simulink model "lsys1"  (R2020b)
settings: Solver=VariableStepAuto  StartTime=0.0  StopTime=10.0  RelTol=1e-3
settings Model: Creator=반달  LastModifiedBy=반달

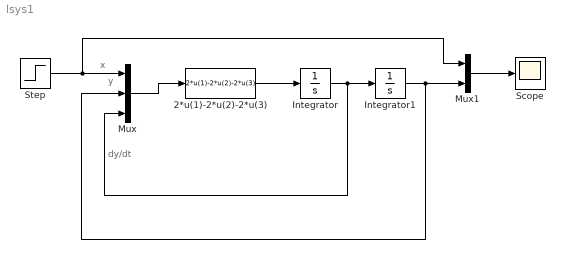
== system lsys1 ==
  note: dy/dt
  note: y
  note: x
  2*u(1)-2*u(2)-2*u(3) : MATLABFcn  MATLABFcn=2*u(1)-2*u(2)-2*u(3)
  Integrator : Integrator
  Integrator1 : Integrator
  Mux : Mux  Inputs=3
  Mux1 : Mux  Inputs=2
  Scope : Scope
  Step : Step  Time=0  SampleTime=0
  wires:
  Step/1 -> Mux1/1, Mux/1
  Mux/1 -> 2*u(1)-2*u(2)-2*u(3)/1
  2*u(1)-2*u(2)-2*u(3)/1 -> Integrator/1
  Integrator/1 -> Mux/3, Integrator1/1
  Integrator1/1 -> Mux/2, Mux1/2
  Mux1/1 -> Scope/1
